simulink model "check_equilibrium"  (R2019b)
settings: Solver=VariableStepAuto  StartTime=0.0  StopTime=10  RelTol=1e-3
values from neighbouring files (symbols this model uses):
  A = [-0.0391932075235  0; 0.0391932075235  -0.0381972328031]    [lin_ss_cont.mat]    (also in script_check_equilibrium.m = [[(-k_1/(2*sqrt(xe1))), 0]; [(k_1/(2*sqrt(xe1))), (-k_2/(2*s)
  B = [0.936765947069  0; 0  0]    [lin_ss_cont.mat]    (also in script_check_equilibrium.m = [[(gamma_1/(2*sqrt(beta_1+gamma_1*ue1))), 0];[0, 0]])
  C = [0 1]    [lin_ss_cont.mat]    (also in script_check_equilibrium.m = [0,1])
  D = [0 0]    [lin_ss_cont.mat]    (also in script_check_equilibrium.m = [0,0])
  h_02 = 10.53    [script_check_equilibrium.m]    (also in script_task_2_linear.m; script_task_2_nonlinear.m)
  ue = [ue1; ue2]    [script_check_equilibrium.m]
  xe1 = (k_2*sqrt(xe2)/k_1)^2    [script_check_equilibrium.m]    (also in script_task_2_linear.m = 24.312; script_task_2_nonlinear.m)
  xe2 = 25.53    [script_check_equilibrium.m]    (also in script_task_2_linear.m = 24.844; script_task_2_nonlinear.m)
  ye = 15    [script_check_equilibrium.m]
settings Model: Creator=NicSch02  LastModifiedBy=NicSch02

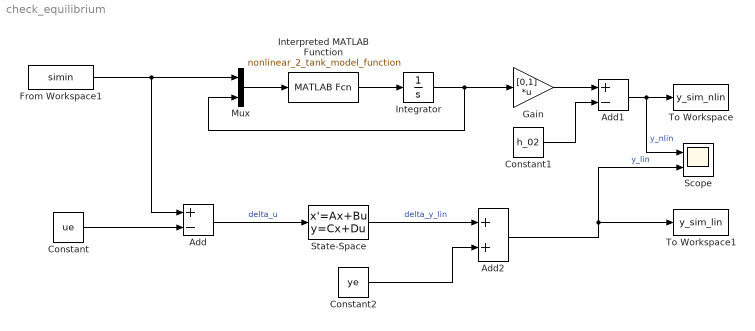
== system check_equilibrium ==
  Add : Sum  Inputs=+-
  Add1 : Sum  Inputs=+-
  Add2 : Sum
  Constant : Constant  Value=ue
  Constant1 : Constant  Value=h_02
  Constant2 : Constant  Value=ye
  From Workspace1 : FromWorkspace  VariableName=simin  SampleTime=0
  Gain : Gain  Gain=[0,1]  Multiplication=Matrix(K*u)
  Integrator : Integrator  InitialCondition=[xe1; xe2;]
  Interpreted MATLAB Function : MATLABFcn  MATLABFcn=nonlinear_2_tank_model_function
  Mux : Mux  Inputs=2
  Scope : Scope  NumInputPorts=2
  State-Space : StateSpace  A=A  B=B  C=C  D=D  InitialCondition=[0; 0]
  To Workspace : ToWorkspace  VariableName=y_sim_nlin  SaveFormat=Structure With Time  SampleTime=-1
  To Workspace1 : ToWorkspace  VariableName=y_sim_lin  SaveFormat=Structure With Time  SampleTime=-1
  wires:
  Add/1 -> State-Space/1  "delta_u"
  From Workspace1/1 -> Add/1, Mux/1
  Constant/1 -> Add/2
  Integrator/1 -> Mux/2, Gain/1
  Interpreted MATLAB Function/1 -> Integrator/1
  Mux/1 -> Interpreted MATLAB Function/1
  Add1/1 -> To Workspace/1, Scope/1  "y_nlin"
  Gain/1 -> Add1/1
  Constant1/1 -> Add1/2
  State-Space/1 -> Add2/1  "delta_y_lin"
  Constant2/1 -> Add2/2
  Add2/1 -> Scope/2, To Workspace1/1  "y_lin"
